simulink model "q2"  (R2017a)
settings: Solver=VariableStepAuto  StartTime=0.0  StopTime=10.0  RelTol=1e-3
values from neighbouring files (symbols this model uses):
  C = [1 0]    [workspace.m]
  fa = -0.35*f2 + 4.45    (= 3.125)    [workspace.m]
  G = [[0.5 1]; [0.5 0.7]]    [workspace.m]
  H1 = [0.2; 0.1]    [workspace.m]
  H2 = [1; 0]    [workspace.m]
settings Model: Creator=arthur  LastModifiedBy=arthur

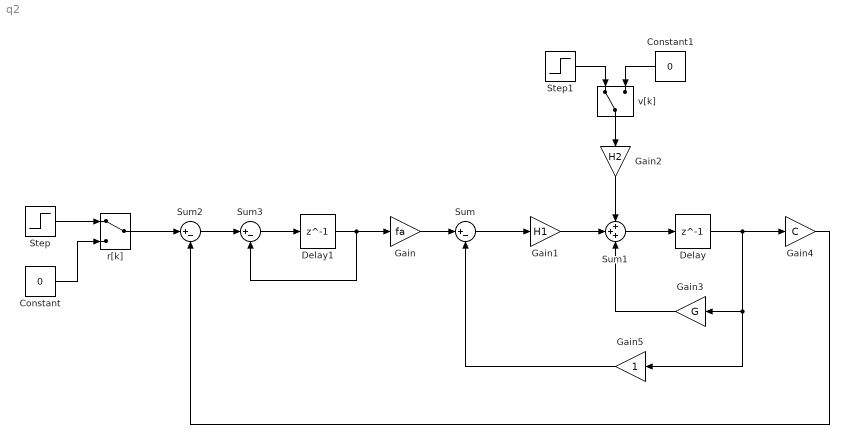
== system q2 ==
  Constant : Constant  Value=0
  Constant1 : Constant  Value=0
  Delay : Delay  DelayLength=1  InitialCondition=0
  Delay1 : Delay  DelayLength=1  InitialCondition=0
  Gain : Gain  Gain=fa
  Gain1 : Gain  Gain=H1
  Gain2 : Gain  Gain=H2
  Gain3 : Gain  Gain=G
  Gain4 : Gain  Gain=C
  Gain5 : Gain
  Step : Step  Time=0  SampleTime=0
  Step1 : Step  Time=0  SampleTime=0
  Sum : Sum  Inputs=|+-
  Sum1 : Sum  Inputs=+++
  Sum2 : Sum  Inputs=|+-
  Sum3 : Sum  Inputs=|+-
  r[k] : ManualSwitch
  v[k] : ManualSwitch
  wires:
  r[k]/1 -> Sum2/1
  Sum2/1 -> Sum3/1
  Sum3/1 -> Delay1/1
  Delay1/1 -> Gain/1, Sum3/2
  Gain/1 -> Sum/1
  Sum/1 -> Gain1/1
  Gain2/1 -> Sum1/1
  Gain1/1 -> Sum1/2
  v[k]/1 -> Gain2/1
  Sum1/1 -> Delay/1
  Delay/1 -> Gain4/1, Gain5/1, Gain3/1
  Gain3/1 -> Sum1/3
  Gain4/1 -> Sum2/2
  Gain5/1 -> Sum/2
  Step1/1 -> v[k]/1
  Step/1 -> r[k]/1
  Constant/1 -> r[k]/2
  Constant1/1 -> v[k]/2
